simulink model "mpc_model_dual_module_allfreq"  (R2019a)
settings: Solver=FixedStepAuto  StartTime=0.0  StopTime=Tfinal  RelTol=1e-3
values from neighbouring files (symbols this model uses):
  A = [-0.0285 -0.0014; -0.0371 -0.1476]    [model.m]
  DCLINK_Cap = 1000e-12    (= 1e-09)    [mpc_model_parameters.m]    (also in mpc_model_parameters_dual_module.m = 0.001)
  FluxPM = MeanInducedVoltagePeak/(2*pi*100)    [mpc_model_parameters.m]    (also in mpc_model_parameters_dual_module.m)
  Inertia = 1e-2    (= 0.01)    [mpc_model_parameters.m]    (also in mpc_model_parameters_dual_module.m)
  iqrated = Trated/(1.5*PolePairs*FluxPM)    [mpc_model_parameters.m]    (also in mpc_model_parameters_dual_module.m)
  Ki = 8    [mpc_model_parameters_dual_module.m]
  Kp = 0.8    [mpc_model_parameters_dual_module.m]
  Ls = 3.5e-3    (= 0.0035)    [MPC_id_iq.m]    (also in mpc_model_parameters.m = 0.00351; mpc_model_parameters_dual_module.m = 0.00343)
  M1_FaultTime = 0.25    [mpc_model_parameters_dual_module.m]
  M2_FaultTime = 20    [mpc_model_parameters_dual_module.m]
  MeanLd = (1/12)*(Module1Phase_A_Ld+Module1Phase_B_Ld+Module1Phase_C_Ld+     Module2Phase_A_Ld+Module2Phase_B_Ld+Module2Phase_C_Ld+     Module3Phase_A_Ld+Module3Phase_B_Ld+Module3Phase_C_Ld+     Module4Phase_A_Ld+Module4Phase_B_Ld+Module4Phase_C_Ld)    [mpc_model_parameters.m]    (also in mpc_model_parameters_dual_module.m)
  MeanLq = (1/12)*(Module1Phase_A_Lq+Module1Phase_B_Lq+Module1Phase_C_Lq+     Module2Phase_A_Lq+Module2Phase_B_Lq+Module2Phase_C_Lq+     Module3Phase_A_Lq+Module3Phase_B_Lq+Module3Phase_C_Lq+     Module4Phase_A_Lq+Module4Phase_B_Lq+Module4Phase_C_Lq)    [mpc_model_parameters.m]    (also in mpc_model_parameters_dual_module.m)
  PI_Frequency = 5000    [mpc_model_parameters_dual_module.m]
  PI_Sat = iqrated*2    [mpc_model_parameters_dual_module.m]
  PI_Ts = 1/PI_Frequency    (= 0.0002)    [mpc_model_parameters_dual_module.m]
  PolePairs = 10    [mpc_model_parameters.m]    (also in mpc_model_parameters_dual_module.m)
  RefModeSelection = 1    [mpc_model_parameters_dual_module.m]
  Rin = 1e-3    (= 0.001)    [mpc_model_parameters.m]    (also in mpc_model_parameters_dual_module.m)
  Rs = 0.531    [Loss_Distribution.m]    (also in MPC_id_iq.m; mpc_model_parameters.m = 0.321; mpc_model_parameters_dual_module.m = 0.539)
  Sampling_time = 1e-6    (= 1e-06)    [mpc_model_parameters.m]    (also in mpc_model_parameters_dual_module.m)
  SpeedRef1 = 50    [mpc_model_parameters.m]    (also in mpc_model_parameters_dual_module.m = 35)
  SpeedRef2 = 100    [mpc_model_parameters.m]    (also in mpc_model_parameters_dual_module.m = 35)
  SpeedRefUpdateTime = 0.25    [mpc_model_parameters.m]    (also in mpc_model_parameters_dual_module.m = 1.75)
  Tload1 = 5    [mpc_model_parameters.m]    (also in mpc_model_parameters_dual_module.m = 30)
  Tload2 = 10    [mpc_model_parameters.m]    (also in mpc_model_parameters_dual_module.m = 63.6619772368)
  TloadUpdateTime = 0.5    [mpc_model_parameters.m]    (also in mpc_model_parameters_dual_module.m)
  Vdc = 50    [mpc_model_parameters.m]    (also in mpc_model_parameters_dual_module.m = 40)
  Vin = Vdc + Rin*(Pout/Vdc)    (= 50.04)    [mpc_model_parameters.m]    (also in mpc_model_parameters_dual_module.m = 40.05)
  ViscousFriction = 1e-3    (= 0.001)    [mpc_model_parameters.m]    (also in mpc_model_parameters_dual_module.m)
undefined symbols (not defined in the file or in its folder): DiscIntNeverNeededParam
libraries: powerlib x27, dspsigops x21, dspswit3 x19, powerlib_meascontrol x10, fl_lib x5, simulink x4, nesl_utility x3, sdl_lib x1
(part 2 of 3)

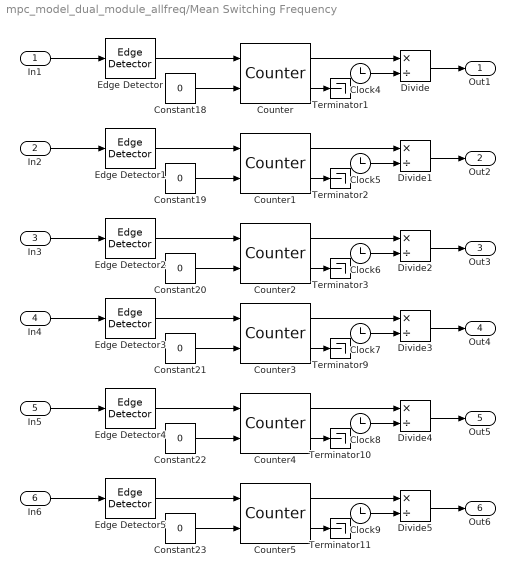
== system mpc_model_dual_module_allfreq/Mean Switching Frequency ==
  In1 : Inport
  In2 : Inport  Port=2
  In3 : Inport  Port=3
  In4 : Inport  Port=4
  In5 : Inport  Port=5
  In6 : Inport  Port=6
  Clock{4..9} (6 alike) : Clock
  Constant{18..23} (6 alike) : Constant  Value=0
  Counter{,1..5} (6 alike) : dspswit3/Counter  Direction=Up  CountEvent=Rising edge  CounterSize=User defined  MaxCount=9999999999999999999  InitialCount=0  Output=Count and Hit  HitValue=32  ResetInput=on  SamplesPerFrame=1  Ts=1  CntDtype=double  HitDtype=Logical
  Divide{,1..5} (6 alike) : Product  Inputs=*/
  Edge Detector{,1..5} (6 alike) : dspswit3/Edge Detector  InputProcessing=Columns as channels (frame based)
      settings: SourceProductName=DSP System Toolbox  SourceProductBaseCode=DS
  Terminator{1..3,9..11} (6 alike) : Terminator
  Out1 : Outport
  Out2 : Outport  Port=2
  Out3 : Outport  Port=3
  Out4 : Outport  Port=4
  Out5 : Outport  Port=5
  Out6 : Outport  Port=6
  wires:
  Counter5/2 -> Terminator11/1
  Divide2/1 -> Out3/1
  Clock8/1 -> Divide4/2
  Counter1/1 -> Divide1/1
  Constant22/1 -> Counter4/2
  Edge Detector5/1 -> Counter5/1
  Counter/2 -> Terminator1/1
  Edge Detector/1 -> Counter/1
  Counter5/1 -> Divide5/1
  Edge Detector2/1 -> Counter2/1
  Edge Detector4/1 -> Counter4/1
  Clock7/1 -> Divide3/2
  Counter4/2 -> Terminator10/1
  Constant19/1 -> Counter1/2
  Counter2/2 -> Terminator3/1
  Clock9/1 -> Divide5/2
  Constant20/1 -> Counter2/2
  Divide5/1 -> Out6/1
  Constant23/1 -> Counter5/2
  Edge Detector1/1 -> Counter1/1
  Counter4/1 -> Divide4/1
  Clock5/1 -> Divide1/2
  Counter3/2 -> Terminator9/1
  Counter2/1 -> Divide2/1
  Constant18/1 -> Counter/2
  In6/1 -> Edge Detector5/1
  Constant21/1 -> Counter3/2
  Counter3/1 -> Divide3/1
  Edge Detector3/1 -> Counter3/1
  Divide3/1 -> Out4/1
  Counter1/2 -> Terminator2/1
  In5/1 -> Edge Detector4/1
  Clock6/1 -> Divide2/2
  Divide/1 -> Out1/1
  Counter/1 -> Divide/1
  Clock4/1 -> Divide/2
  Divide4/1 -> Out5/1
  In4/1 -> Edge Detector3/1
  In2/1 -> Edge Detector1/1
  Divide1/1 -> Out2/1
  In3/1 -> Edge Detector2/1
  In1/1 -> Edge Detector/1

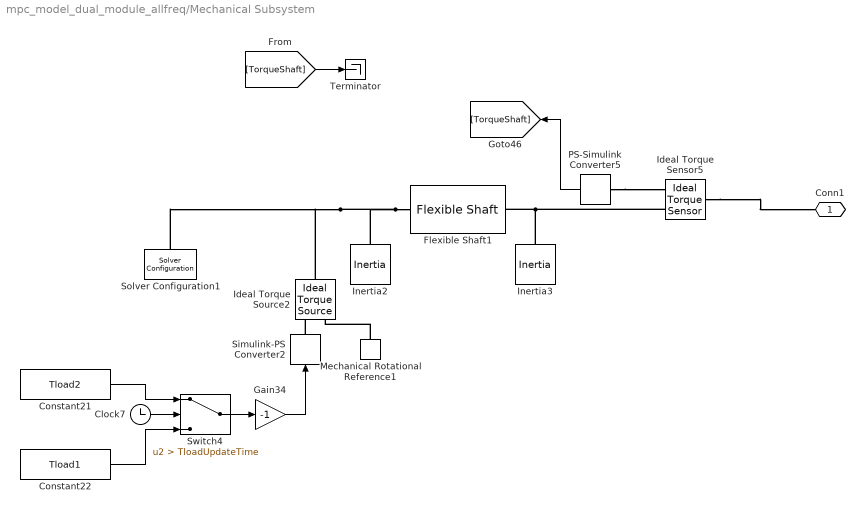
== system mpc_model_dual_module_allfreq/Mechanical Subsystem ==
  Clock7 : Clock
  Constant21 : Constant  Value=Tload2
  Constant22 : Constant  Value=Tload1
  Flexible Shaft1 : sdl_lib/Couplings & Drives/Flexible Shaft  modelTransverse=simscape.enum.onoff.off  parameterization=1  n_segments=10  shaft_stiffness=MechanicalShaftStiffness N*m/rad  shaft_inertia=MechanicalShaftInertia kg*m^2  length=1 m  eiIN=5e5 m^4*Pa  rhoaIN=19 kg/m  shaft_construction=1  diameter_outer=0.075 m  diameter_inner=0.05 m  density=7.8e+3 kg/m^3  shear_modulus=7.93e+10 Pa  elastic_modulus=200e9 Pa  damping_ratio=MechanicalShaftDampingRatio  mu_visc=[ 0 0 ] N*m/(rad/s)  boundaryC=sdl.enum.shaftSupport.clamp  KtransC_row=[10000000, 10000000] N/m  KrotC_row=[10000000, 10000000] N*m/rad  boundaryR=sdl.enum.shaftSupport.clamp  KtransR_row=[10000000, 10000000] N/m  KrotR_row=[10000000, 10000000] N*m/rad  alpha=10 1/s  beta=1e-8 s  d_bearing_trans=[0, 0] N/(m/s)  d_bearing_rotation=[0, 0] N*m/(rad/s)  noDisk=sdl.enum.shaftDisks.none  zDisk=0.5 m  mDiskIN=2 kg  IdDiskIN=0.025 kg*m^2  IpDiskIN=0.050 kg*m^2  offsetMR=[.01, .01] m*kg  offsetMassLocation=[.33, .67] m  offsetMR_initialAngleIN=[0, pi] rad  AnalysisMethod=sdl.enum.bendingAnalysisMethod.LumpedMass  ModeInputMethod=sdl.enum.modeInputMethod.SimscapeDetermined  numModesIn=6  OmegaNom=100 rpm  dw=5 rad/s  dwRefineFactor=1e-4  wMax=50000 rad/s  dz=0.01 m  userMode_w=[162, 162, 649, 649, 1460, 1460, 2596, 2596] rad/s  userMode_z=[0 : 0.1 : 1] m  userMode_shape=[0, 0, 0, 0, 0, 0, 0, 0, 0, 0, 0, 0, 0, 0, 0, 0; .309, 0, 0, .309, .5878, 0, 0, .5878, .809, 0, 0, .809, .9511, 0, 0, .9511; .5878, 0, 0, .5878, .9511, 0, 0, .9511, .9511, 0, 0, .9511, .5878, 0, 0, .5878; .809, 0, 0, .809, .9511, 0, 0, .9511, .309, 0, 0, .309, -.5878, 0, 0, -.5878; .9511, 0, 0, .9511, .5878, 0, 0, .5878, -.5878, 0, 0, -.5878, -.9511, 0, 0, -.9511; 1, 0, 0, 1, 0, 0, 0, 0, -1, 0, 0, -1, 0, 0, 0, 0; .9511, 0, 0, .9511, -.5878, 0, 0, -.5878, -.5878, 0, 0, -.5878, .9511, 0, 0, .9511; .809, 0, 0, .809, -.9511, 0, 0, -.9511, .309, 0, 0, .309, .5878, 0, 0, .5878; .5878, 0, 0, .5878, -.9511, 0, 0, -.9511, .9511, 0, 0, .9511, -.5878, 0, 0, -.5878; .309, 0, 0, .309, -.5878, 0, 0, -.5878, .809, 0, 0, .809, -.9511, 0, 0, -.9511; 0, 0, 0, 0, 0, 0, 0, 0, 0, 0, 0, 0, 0, 0, 0, 0]  initial_deflection=0 rad  initial_velocity=0 rpm
      settings: SourceProductName=Simscape Driveline  SourceProductBaseCode=LD
  Gain34 : Gain  Gain=-1
  Ideal Torque Sensor5 : fl_lib/Mechanical/Mechanical Sensors/Ideal Torque Sensor
  Ideal Torque Source2 : fl_lib/Mechanical/Mechanical Sources/Ideal Torque Source
  Inertia2 : fl_lib/Mechanical/Rotational Elements/Inertia  inertia=MechanicalInertia1 kg*m^2  w_specify=off  w_priority=High  w=0 rad/s  w_nominal_specify=off  w_nominal_unit=rad/s  w_nominal_value=1  t_specify=off  t_priority=None  t=0 N*m  t_nominal_specify=off  t_nominal_unit=N*m  t_nominal_value=1
  Inertia3 : fl_lib/Mechanical/Rotational Elements/Inertia  inertia=MechanicalInertia1 kg*m^2  w_specify=off  w_priority=High  w=0 rad/s  w_nominal_specify=off  w_nominal_unit=rad/s  w_nominal_value=1  t_specify=off  t_priority=None  t=0 N*m  t_nominal_specify=off  t_nominal_unit=N*m  t_nominal_value=1
  Mechanical Rotational Reference1 : fl_lib/Mechanical/Rotational Elements/Mechanical Rotational Reference
  PS-Simulink Converter5 : nesl_utility/PS-Simulink Converter  PhysicalDomain=network_engine_domain  SubClassName=ps_output  LeftPortType=input  RightPortType=output  PseudoPeriodic=off  Frequencies=[]  Unit=1  AffineConversion=off
  Simulink-PS Converter2 : nesl_utility/Simulink-PS Converter  PhysicalDomain=network_engine_domain  SubClassName=ps_input  LeftPortType=input  RightPortType=output  PseudoPeriodic=off  Frequencies=[]  NoiseDistribution=none  NoiseParameters=[]  Unit=1  AffineConversion=off  FilteringAndDerivatives=zero  SimscapeFilterOrder=1  InputFilterTimeConstant=0.001  UdotUserProvided=1
  Solver Configuration1 : nesl_utility/Solver Configuration  PhysicalDomain=network_engine_domain  SubClassName=solver  LeftPortType=input  RightPortType=generic  Tones=[]  Harmonics=[]  SimulateNoise=off  Profile=off  UseLocalSampling=off  EnableSwitchedLinearOptims=on  FrequencyDomain=off  UseCCode=off  RelTol=0.001  AbsTol=1e-06  MinStep=1e-09  ToWorkspace=off  RevertToSquareIcSolve=off  NumHomotopyIterations=100  PhasorMode=off  PhasorModeNumHarmonics=1  DoDC=off  ResidualTolerance=1e-09  UseLocalSolver=off  LocalSolverChoice=NE_BACKWARD_EULER_ADVANCER  LocalSolverSampleTime=0.001  DoFixedCost=off  MaxNonlinIter=3  MaxModeIter=2  LinearAlgebra=Sparse  EquationFormulation=NE_TIME_EF  DelaysMemoryBudget=1024  AutomaticFiltering=on  FilteringTimeConstant=0.001  PartitionStorageMethod=AS_NEEDED  PartitionMemoryBudget=1024  PartitionMethod=FAST
  Switch4 : Switch  Criteria=u2 > Threshold  Threshold=TloadUpdateTime
  Terminator : Terminator
  Conn1 : PMIOPort  Side=Left
  wires:
  Clock7/1 -> Switch4/2
  Constant21/1 -> Switch4/1
  Gain34/1 -> Simulink-PS Converter2/1
  PS-Simulink Converter5/1 -> [TorqueShaft]
  Switch4/1 -> Gain34/1
  Constant22/1 -> Switch4/3
  [TorqueShaft] -> Terminator/1
  connections:
  Flexible Shaft1/LConn1 -- Inertia2/LConn1 -- Solver Configuration1/RConn1 -- Ideal Torque Source2/LConn1
  Ideal Torque Sensor5/LConn1 -- Conn1/RConn1
  Ideal Torque Sensor5/RConn1 -- Inertia3/LConn1 -- Flexible Shaft1/RConn1
  Simulink-PS Converter2/RConn1 -- Ideal Torque Source2/RConn1
  Mechanical Rotational Reference1/LConn1 -- Ideal Torque Source2/RConn2
  PS-Simulink Converter5/LConn1 -- Ideal Torque Sensor5/RConn2

== matlab function mpc_model_dual_module_allfreq/MATLAB Function3 ==
  data: M1_copperloss output; M2_copperloss output; M1_magneticloss output; M2_magneticloss output; iqref input; M1_iqref output; M1_idref output; M2_iqref output; M2_idref output; Rs input; M1_FaultTime input; clock input; Ls input; ElectricalAngle input; M1_iqref_prev input; M1_idref_prev input; M2_iqref_prev input; M2_idref_prev input; M1_Iq_Opt_Proportional_prev input; M1_Id_Opt_Proportional_prev input; M2_Iq_Opt_Proportional_prev input; M2_Id_Opt_Proportional_prev input; ElectricalSpeed input; FluxPM input; pulse input; M1_Iq_Opt_Proportional output; M1_Id_Opt_Proportional output; M2_Iq_Opt_Proportional output; M2_Id_Opt_Proportional output; weight output; M1_lossfactor output; M2_lossfactor output; M1_lossfactor_prev input; M2_lossfactor_prev input
function [M1_copperloss,M2_copperloss,M1_magneticloss,M2_magneticloss,M1_iqref, M1_idref, M2_iqref, M2_idref,M1_Iq_Opt_Proportional,M1_Id_Opt_Proportional,M2_Iq_Opt_Proportional,M2_Id_Opt_Proportional,weight,M1_lossfactor,M2_lossfactor] = fcn(iqref, Rs, M1_FaultTime, clock, Ls, ElectricalAngle,M1_iqref_prev, M1_idref_prev, M2_iqref_prev, M2_idref_prev, M1_Iq_Opt_Proportional_prev, M1_Id_Opt_Proportional_prev, M2_Iq_Opt_Proportional_prev, M2_Id_Opt_Proportional_prev, ElectricalSpeed, FluxPM, pulse,M1_lossfactor_prev,M2_lossfactor_prev)

iqrated = 11.7362;
optimizationstep = 100;

% M2_iqref = iqref-M1_iqs;
M1_iqref_hyp = zeros(1,optimizationstep+1);
M2_iqref_hyp = zeros(1,optimizationstep+1);
M1_idref_hyp = zeros(1,optimizationstep+1);
M2_idref_hyp = zeros(1,optimizationstep+1);

M1_copper_loss = zeros(1,optimizationstep+1);
M2_copper_loss = zeros(1,optimizationstep+1);
M1_magnetic_loss = zeros(1,optimizationstep+1);
M2_magnetic_loss = zeros(1,optimizationstep+1);
Total_copper_loss = zeros(1,optimizationstep+1);
Total_magnetic_loss = zeros(1,optimizationstep+1);
cost = zeros(1,optimizationstep+1);
MinLossIndex = 0;

M1_Possible_Iq = zeros(1,optimizationstep+1);
M1_Possible_Id = zeros(1,optimizationstep+1);
M2_Possible_Iq = zeros(1,optimizationstep+1);
M2_Possible_Id = zeros(1,optimizationstep+1);

M1_magneticloss = 0;
M2_magneticloss = 0;

M1_copperloss = 0;
M2_copperloss = 0;

cfe = 1.15;
lambda = 1.15;
weight = 1;

% if(clock>M1_FaultTime)
if(iqref>iqrated)
    M1_lossfactor = 1;
    M2_lossfactor = 1;    
else
    M1_lossfactor = 1;
    M2_lossfactor = 1;    
end



% % % if(iqref>iqrated)
% % %     M1_lossfactor = 3;
% % %     M2_lossfactor = 2;
% % % else
% % %     M1_lossfactor = 1;
% % %     M2_lossfactor = 1;
% % % end

if(pulse==1)
    for i = 0:optimizationstep
        if(clock>M1_FaultTime)
% % % % %             M1_Possible_Iq(i+1) =  2/3*sin(2*pi/3)*(1+cos(2*ElectricalAngle+pi));
% % % % %             M1_Possible_Id(i+1) =  2/3*sin(2*pi/3)*(sin(2*ElectricalAngle+pi));
% % % % %             M2_Possible_Iq(i+1) = 1;
% % % % %             M2_Possible_Id(i+1) = 0;
            if(iqref>iqrated)
                M1_Possible_Iq(i+1) =  2*2/3*sin(2*pi/3)*(1+cos(2*ElectricalAngle+pi));
                M1_Possible_Id(i+1) =  2*2/3*sin(2*pi/3)*(sin(2*ElectricalAngle+pi));
                M2_Possible_Iq(i+1) = 1;
                M2_Possible_Id(i+1) = 0;
            else
                M1_Possible_Iq(i+1) =  1*2/3*sin(2*pi/3)*(1+cos(2*ElectricalAngle+pi));
                M1_Possible_Id(i+1) =  1*2/3*sin(2*pi/3)*(sin(2*ElectricalAngle+pi));
                M2_Possible_Iq(i+1) = 1;
                M2_Possible_Id(i+1) = 0;
            end
        else
            M1_Possible_Iq(i+1) = 1;
            M1_Possible_Id(i+1) = 0;
            M2_Possible_Iq(i+1) = 1;
            M2_Possible_Id(i+1) = 0;
        end
        
%         if(clock>M1_FaultTime)
            M1_iqref_hyp(i+1) = (1/optimizationstep*i)*iqref*M1_Possible_Iq(i+1);
            M1_idref_hyp(i+1) = (1/optimizationstep*i)*iqref*M1_Possible_Id(i+1);

            M2_iqref_hyp(i+1) = iqref - M1_iqref_hyp(i+1);
            if(iqref>iqrated)
%                weight = 4.2605;
                 weight = abs(iqrated-M1_iqref_hyp(i+1))/iqrated/10;
            else
%                weight = 1;
            end
            

            
            loss_protection  = 0;
            
            if(M2_iqref_hyp(i+1)>1.5*iqrated)
%                 loss_protection = 100;
            end
            weight = 1;
            
%             M1_lossfactor = 2/3;
%             M2_lossfactor = 1;

            
%         else
%             M1_iqref_hyp(i+1) = (1/optimizationstep*i)*iqref;
%             M2_iqref_hyp(i+1) = (1-1/optimizationstep*i)*iqref;
%             
%         end
        
        M1_d_axis_flux = Ls*M1_idref_hyp(i+1)+FluxPM;
        M1_q_axis_flux = Ls*M1_iqref_hyp(i+1);
        M2_d_axis_flux = Ls*M2_idref_hyp(i+1)+FluxPM;
        M2_q_axis_flux = Ls*M2_iqref_hyp(i+1);

        M1_copper_loss(i+1) = 1.5*Rs*(M1_iqref_hyp(i+1)^2+M1_idref_hyp(i+1)^2);
        M2_copper_loss(i+1) = 1.5*Rs*(M2_iqref_hyp(i+1)^2+M2_idref_hyp(i+1)^2);
        
%         M1_magnetic_loss(i+1) = cfe*power(abs(ElectricalSpeed),lambda)*(M1_d_axis_flux^2+M1_q_axis_flux^2);
%         M2_magnetic_loss(i+1) = cfe*power(abs(ElectricalSpeed),lambda)*(M2_d_axis_flux^2+M2_q_axis_flux^2);
        
        Total_magnetic_loss(i+1) = M1_magnetic_loss(i+1)+ M2_magnetic_loss(i+1);
%         Total_copper_loss(i+1) = M1_copper_loss(i+1)*weight+M2_copper_loss(i+1);
        Total_copper_loss(i+1) = M1_copper_loss(i+1)*M1_lossfactor_prev+M2_copper_loss(i+1)*M2_lossfactor_prev;
        
%         cost(i+1) = Total_copper_loss(i+1) + 0*Total_magnetic_loss(i+1) + loss_protection;    % +100000*(M1_idref_hyp(i+1)^2);%;+200000000000*(M1_idref_hyp(i+1)^2);
        cost(i+1) = Total_copper_loss(i+1);    % +100000*(M1_idref_hyp(i+1)^2);%;+200000000000*(M1_idref_hyp(i+1)^2);
        
        
    end
    
    [MinLossValue,MinLossIndex] = min(cost);
    if(clock>M1_FaultTime)
        M1_Iq_Opt_Proportional = iqref*0.5*2/7*(1+cos(2*ElectricalAngle+pi));
        M1_Id_Opt_Proportional = iqref*0.5*2/7*(sin(2*ElectricalAngle+pi));
        M2_Iq_Opt_Proportional = iqref*0.5*(5/7-2/7*cos(2*ElectricalAngle+pi));
        M2_Id_Opt_Proportional = 0;
    else
        M1_Iq_Opt_Proportional = iqref*0.5;
        M1_Id_Opt_Proportional = 0;
        M2_Iq_Opt_Proportional = iqref*0.5;
        M2_Id_Opt_Proportional = 0;
    end
    
    M1_iqref = M1_iqref_hyp(MinLossIndex);
    M1_idref = M1_idref_hyp(MinLossIndex);
    
    M2_iqref = M2_iqref_hyp(MinLossIndex);
    M2_idref = M2_idref_hyp(MinLossIndex);
    
%     if(M2_iqref>iqrated)
% %             M1_lossfactor = 2/3;
%         M2_lossfactor = M2_lossfactor_prev+0.01;
%     else
%         if(clock>M1_FaultTime)
%         M2_lossfactor = M2_lossfactor_prev-0.01;
%         end
%     end
%     
    M1_magneticloss = M1_magnetic_loss(MinLossIndex);
    M2_magneticloss = M2_magnetic_loss(MinLossIndex);
    
    M1_copperloss = M1_copper_loss(MinLossIndex);
    M2_copperloss = M2_copper_loss(MinLossIndex);

    
else
    M1_iqref = M1_iqref_prev;
    M1_idref = M1_idref_prev;
    
    M2_iqref = M2_iqref_prev;
    M2_idref = M2_idref_prev;
    
    M1_Iq_Opt_Proportional = M1_Iq_Opt_Proportional_prev;
    M1_Id_Opt_Proportional = M1_Id_Opt_Proportional_prev;
    M2_Iq_Opt_Proportional = M2_Iq_Opt_Proportional_prev;
    M2_Id_Opt_Proportional = M2_Id_Opt_Proportional_prev;    
    

    
end

== matlab function mpc_model_dual_module_allfreq/MATLAB Function ==
  data: d input; a output; q input; zero input; b output; c output; angle input
function [a,b,c] = fcn(d,q,zero,angle)

a = sin(angle)          *d  + cos(angle)        *q + 1*zero;
b = sin(angle-2*pi/3)   *d  + cos(angle-2*pi/3) *q + 1*zero;
c = sin(angle+2*pi/3)   *d  + cos(angle+2*pi/3) *q + 1*zero;

== matlab function mpc_model_dual_module_allfreq/M2 Prediction ==
  data: DutyA output; DutyB output; DutyC output; iqref input; idref input; IdMeasured input; IqMeasured input; Ls input; Rs input; PolePairs input; wref input; ShaftAngularSpeed input; ShaftAngularSpeed_prev input; FluxPM input; Vdc input; ElectricalAngle input; InterruptPulse input; DutyA_prev input; DutyB_prev input; DutyC_prev input; SimulationClock input; FaultOccuranceTime input; FswSelected_prev input; FswSelected output; IqRipplePrediction output; IqRipplePrediction_prev input; Speed_Error_prev input; Speed_Error output; Vds_Optimum output; Vqs_Optimum output; Vds_Optimum_prev input; Vqs_Optimum_prev input; fsw_phase input; M1_fsw input; M2_fsw_prev input; M1_int_moment input; M2_int_moment input; filter_out output; filter_out_prev input; IdPrediction_1_array output; IqPrediction_1_array output; IdPrediction_2_array output; IqPrediction_2_array output
function [DutyA, DutyB, DutyC, FswSelected, IqRipplePrediction,Speed_Error,Vds_Optimum,Vqs_Optimum,filter_out,IdPrediction_1_array,IqPrediction_1_array,IdPrediction_2_array,IqPrediction_2_array] = fcn(iqref,idref,IdMeasured, IqMeasured,  Ls, Rs,PolePairs,wref, ShaftAngularSpeed, ShaftAngularSpeed_prev, FluxPM,Vdc,ElectricalAngle,InterruptPulse,DutyA_prev, DutyB_prev, DutyC_prev, SimulationClock,FaultOccuranceTime,FswSelected_prev, IqRipplePrediction_prev,Speed_Error_prev,Vds_Optimum_prev,Vqs_Optimum_prev, fsw_phase, M1_fsw, M2_fsw_prev,M1_int_moment, M2_int_moment,filter_out_prev)
Ld = Ls;
Lq = Ls;
Iq_Rated = 11.7362; %this is the rated value of the IqMeasured



% cost = zeros(1,8);
% VdPrediction_1 = zeros(1,8);
% VqPrediction_1 = zeros(1,8);
% FswOptions = [5000; 10000; 15000; 20000; 25000; 30000; 35000; 40000];
FswMax = 10000;
FswOptions = 1000:1000:FswMax;
cost = zeros(1,numel(FswOptions));
% VdPrediction_1 = zeros(1,numel(FswOptions));
% VqPrediction_1 = zeros(1,numel(FswOptions));
Vd_est_1 = zeros(1,numel(FswOptions));
Vq_est_1 = zeros(1,numel(FswOptions));
% Vd_est_2 = zeros(1,numel(FswOptions));
% Vq_est_2 = zeros(1,numel(FswOptions));
VdPrediction_2 = zeros(1,numel(FswOptions));
VqPrediction_2 = zeros(1,numel(FswOptions));
IqRipplePredictionArray_1 = zeros(1,numel(FswOptions));
IqRipplePredictionArray_2 = zeros(1,numel(FswOptions));
VoltageDuring_T1_1 = zeros(1,numel(FswOptions));
VoltageDuring_T2_1 = zeros(1,numel(FswOptions));
VoltageDuring_T0_1 = zeros(1,numel(FswOptions));
VoltageDuring_T1_2 = zeros(1,numel(FswOptions));
VoltageDuring_T2_2 = zeros(1,numel(FswOptions));
VoltageDuring_T0_2 = zeros(1,numel(FswOptions));
MagnitudePrediction_1 = zeros(1,numel(FswOptions));
MagnitudePrediction_2 = zeros(1,numel(FswOptions));

SvpwmT1Prediction_1 =  zeros(1,numel(FswOptions));
SvpwmT2Prediction_1 =  zeros(1,numel(FswOptions));
SvpwmT0Prediction_1 =  zeros(1,numel(FswOptions));

SvpwmT1Prediction_2 =  zeros(1,numel(FswOptions));
SvpwmT2Prediction_2 =  zeros(1,numel(FswOptions));
SvpwmT0Prediction_2 =  zeros(1,numel(FswOptions));

ValfaPrediction_1 = zeros(1,numel(FswOptions)); 
VbetaPrediction_1 = zeros(1,numel(FswOptions)); 
ValfaPrediction_2 = zeros(1,numel(FswOptions)); 
VbetaPrediction_2 = zeros(1,numel(FswOptions)); 
maPrediction_1 = zeros(1,numel(FswOptions)); 
maPrediction_2 = zeros(1,numel(FswOptions));

IqDelta_Prediction_During_T1_1 =  zeros(1,numel(FswOptions));
IqDelta_Prediction_During_T2_1 =  zeros(1,numel(FswOptions));
IqDelta_Prediction_During_T0_1 =  zeros(1,numel(FswOptions));
IqDelta_Prediction_During_T1_2 =  zeros(1,numel(FswOptions));
IqDelta_Prediction_During_T2_2 =  zeros(1,numel(FswOptions));
IqDelta_Prediction_During_T0_2 =  zeros(1,numel(FswOptions));
VoltageVectorAnglePredictionMod_1 = zeros(1,numel(FswOptions));
VoltageVectorAnglePrediction_1 = zeros(1,numel(FswOptions));
VoltageVectorAnglePredictionMod_2 = zeros(1,numel(FswOptions));
VoltageVectorAnglePrediction_2 = zeros(1,numel(FswOptions));

IdPrediction_1_array = zeros(1,numel(FswOptions));
IqPrediction_1_array = zeros(1,numel(FswOptions));
IdPrediction_2_array = zeros(1,numel(FswOptions));
IqPrediction_2_array = zeros(1,numel(FswOptions));

Vd_Vq_Kp = 10;
Vd_Vq_Ki = 1;

MinimumCostValue = 1e20;
MinimumCostIndex = -1;

p1 = zeros(1,numel(FswOptions));
p2 = zeros(1,numel(FswOptions));
p3 = zeros(1,numel(FswOptions));
p4 = zeros(1,numel(FswOptions));
p5 = zeros(1,numel(FswOptions));
p6 = zeros(1,numel(FswOptions));


M1_Next_Int_Moment = M1_int_moment + 1/M1_fsw;

% IqRippleCoeff = 100000;
% IqRefCoeff = 10000;
% IdRefCoeff = 15;
% FswCoeff = 1250;
% FswCoeff = ones(1,numel(FswOptions))*1050;

IqRippleCoeff = 1000000;
IqRefCoeff = 1000000;
IdRefCoeff = 1000000;
% % FswCoeff = 2000;
% % FswInertiaCoeff = 500;
FswPhaseCoeff = 5000;

FswCoeff = 1250/10;
FswInertiaCoeff = 750;

M1fsw_M2fsw_PhaseDifference = M2_int_moment - M1_int_moment;


Iq_1_Method1 = 0;
Id_1_Method1 = 0;
Iq_2_Method1 = 0;
Id_2_Method1 = 0;
Kp = 0.35;
Ki = 50;
Ts_PI = 1/40000;
OptimizeForFsws = 0;
DifferentFswCost = 0;
if(FswSelected_prev<=0)
    FswSelected_prev = 1000;
end
% % % % % if(FswSelected_prev==1000)
% % % % %     OptimizeForFsws = 1:1:2;
% % % % % else if(FswSelected_prev==10000)
% % % % %      OptimizeForFsws = 9:1:10;
% % % % %     else
% % % % %         OptimizeForFsws = (FswSelected_prev/1000-1):1:(FswSelected_prev/1000+1);
% % % % %     end
% % % % % end

% % % % % % % % % if((FswSelected_prev==1000)||(FswSelected_prev==2000))
% % % % % % % % %     OptimizeForFsws = 1:1:5;
% % % % % % % % % else if((FswSelected_prev==10000)||(FswSelected_prev==9000))
% % % % % % % % %      OptimizeForFsws = 5:1:10;
% % % % % % % % %     else
% % % % % % % % %         OptimizeForFsws = (FswSelected_prev/1000-2):1:(FswSelected_prev/1000+2);
% % % % % % % % %     end
% % % % % % % % % end

if(FswSelected_prev==1000)
    OptimizeForFsws = 1:1:2;
else if(FswSelected_prev==10000)
     OptimizeForFsws = 9:1:10;
    else
        OptimizeForFsws = (FswSelected_prev/1000-1):1:(FswSelected_prev/1000+1);
    end
end


M1fsw_M2fsw_PhaseDifference_prediction = 0;


Speed_Error =  wref-ShaftAngularSpeed;
Speed_Error_RPM = Speed_Error/(2*pi)*60;

% deriv_speed = (ShaftAngularSpeed - ShaftAngularSpeed_prev)* FswSelected_prev;

if((abs(Speed_Error_RPM)>5)||(abs(filter_out_prev/100)>5))
    %         OptimizeForFsws(3) = 10;
    %         OptimizeForFsws(2) = 9;
    % IqRippleCoeff = 100000;
    IqRefCoeff = 1000000*100;
    IdRefCoeff = 1000000*100;
    FswPhaseCoeff = 0;
    % FswCoeff = 2500/5;
else
    IqRippleCoeff = 100000;
    IqRefCoeff = 1000000;
    IdRefCoeff = 1000000;
    FswPhaseCoeff = 5000;    
%     FswCoeff = 2000;
end


% y = y_prev + Kp*(u-u_prev)+Ts/2*Ki*(u+u_prev);
if(InterruptPulse==1)
    Speed_Error =  wref-ShaftAngularSpeed;
    Speed_Error_RPM =  Speed_Error/(2*pi)*60;
    
    
    filter_out = filter_out_prev + Speed_Error_RPM;
    filter_out = filter_out - filter_out/100;
        
%     iqref = iqref_prev + Kp*(Speed_Error-Speed_Error_prev)+Ts_PI/2*Ki*((Speed_Error+Speed_Error_prev));
% 
%     if(abs(iqref)>(2*Iq_Rated))
%         if(iqref>0)
%             iqref = (2*Iq_Rated);
%         else
%             iqref = -(2*Iq_Rated);
%         end
%     end
    for i = 1:numel(FswOptions)
%     for i = OptimizeForFsws(1):OptimizeForFsws(end)

        IdPrediction_1 = IdMeasured + (0.5/FswSelected_prev + 0.5/FswOptions(i))*(Vds_Optimum_prev/Ld-Rs/Ld*IdMeasured+Lq/Ld*PolePairs*ShaftAngularSpeed*IqMeasured);
        IqPrediction_1 = IqMeasured + (0.5/FswSelected_prev + 0.5/FswOptions(i))*(Vqs_Optimum_prev/Lq-Rs/Lq*IqMeasured-Ld/Lq*PolePairs*ShaftAngularSpeed*IdMeasured-FluxPM*PolePairs*ShaftAngularSpeed/Lq);
        
                
        IdPrediction_1_array(i) = IdPrediction_1;
        IqPrediction_1_array(i) = IqPrediction_1;

        M2_Next_Int_Moment = M2_int_moment + 1/FswOptions(i);
%         if(FswOptions(i) == M1_fsw)
%             if (((abs(M2_Next_Int_Moment-M1_Next_Int_Moment))*M1_fsw) > 0.74) && (((abs(M2_Next_Int_Moment-M1_Next_Int_Moment))*M1_fsw) < 0.76)
%                 
%             else
%                 
%                 FswCoeff(i) = 1250*3;
% %                 IqRippleCoeff = 100000;
%             end
%             DifferentFswCost = 0;            
%         else
%             FswCoeff(i) = 1250;
%             DifferentFswCost = 1500;
%             IqRippleCoeff = 100000;
%         end        
        
        Vd_Vq_Kp = Ls/(2)*FswOptions(i);
        Vd_Vq_Ki = Rs/Ls;
        
        Vd_est_1(i) = Vd_Vq_Kp * (idref-IdPrediction_1) * ( 1 + Vd_Vq_Ki / FswOptions(i) ) + IdMeasured - PolePairs*ShaftAngularSpeed*Ls*IqPrediction_1;
        Vq_est_1(i) = Vd_Vq_Kp * (iqref-IqPrediction_1) * ( 1 + Vd_Vq_Ki / FswOptions(i) ) + IqMeasured + PolePairs*ShaftAngularSpeed*(Ls*IdPrediction_1 + FluxPM);

        
     
        
        %% second prediction
        
%         M1fsw_M2fsw_PhaseDifference_prediction = - 1/M1_fsw + M1fsw_M2fsw_PhaseDifference + 1/FswOptions(i);        
        
        M1fsw_M2fsw_PhaseDifference_prediction = (M1fsw_M2fsw_PhaseDifference*FswOptions(i)-0.25)^2;
        
        MagnitudePrediction_2(i) = sqrt(Vd_est_1(i)^2+Vq_est_1(i)^2);
        
        ValfaPrediction_2(i) = sin(ElectricalAngle)*Vd_est_1(i)+cos(ElectricalAngle)*Vq_est_1(i);
        VbetaPrediction_2(i) =-cos(ElectricalAngle)*Vd_est_1(i)+sin(ElectricalAngle)*Vq_est_1(i);      
        
        VoltageVectorAnglePrediction_2(i) = atan2(VbetaPrediction_2(i),ValfaPrediction_2(i))+4*pi;%(PolePairs*ShaftAngularSpeed/FswOptions(i));
        VoltageVectorAnglePredictionMod_2(i) = mod(VoltageVectorAnglePrediction_2(i),pi/3);   
        
        maPrediction_2(i) = MagnitudePrediction_2(i)/(Vdc/sqrt(3)); 
        
        SvpwmT1Prediction_2(i) = (1/FswOptions(i))*maPrediction_2(i)*sin(pi/3-VoltageVectorAnglePredictionMod_2(i));
        SvpwmT2Prediction_2(i) = (1/FswOptions(i))*maPrediction_2(i)*sin(VoltageVectorAnglePredictionMod_2(i));
        SvpwmT0Prediction_2(i) = (1/FswOptions(i))-SvpwmT1Prediction_2(i)-SvpwmT2Prediction_2(i); 
        
        VoltageDuring_T1_2(i) = 2/3*Vdc-MagnitudePrediction_2(i);
        VoltageDuring_T2_2(i) = 2/3*Vdc-MagnitudePrediction_2(i);
        VoltageDuring_T0_2(i) = -MagnitudePrediction_2(i);
        
        IqDelta_Prediction_During_T1_2(i) = -VoltageDuring_T1_2(i)*SvpwmT1Prediction_2(i)/Ls;
        IqDelta_Prediction_During_T2_2(i) = -VoltageDuring_T2_2(i)*SvpwmT2Prediction_2(i)/Ls;
        IqDelta_Prediction_During_T0_2(i) = VoltageDuring_T0_2(i)*SvpwmT0Prediction_2(i)/Ls;        
        
        IqRipplePredictionArray_2(i) = IqDelta_Prediction_During_T1_2(i)+IqDelta_Prediction_During_T2_2(i)+IqDelta_Prediction_During_T0_2(i);
        
        IdPrediction_2 = IdPrediction_1 + (1/FswOptions(i))*(Vd_est_1(i)/Ld-Rs/Ld*IdPrediction_1+Lq/Ld*PolePairs*ShaftAngularSpeed*IqPrediction_1);
        IqPrediction_2 = IqPrediction_1 + (1/FswOptions(i))*(Vq_est_1(i)/Lq-Rs/Lq*IqPrediction_1-Ld/Lq*PolePairs*ShaftAngularSpeed*IdPrediction_1-FluxPM*PolePairs*ShaftAngularSpeed/Lq);                
        
        IdPrediction_2_array(i) = IdPrediction_2;
        IqPrediction_2_array(i) = IqPrediction_2;
        

        ProtectionConstant = 0;
        
        
% % %         cost(i) = M1fsw_M2fsw_PhaseDifference_prediction * 10000/4 + 0*50000*( abs(M1fsw_M2fsw_PhaseDifference_prediction) *  M1_fsw - .25)^2 + DifferentFswCost + 0*500*((FswOptions(i)-M1_fsw)/FswMax)^2+(IqRipplePredictionArray_2(i)/Iq_Rated)^2*IqRippleCoeff+IqRefCoeff*((iqref-IqPrediction_2)/Iq_Rated)^2+((idref-IdPrediction_2)/Iq_Rated)^2*IdRefCoeff+ProtectionConstant+FswOptions(i)/FswMax*FswCoeff(i);%+IqRipplePrediction_prev^2*100000000;
%         cost(i) = abs(M2_fsw_prev-FswOptions(i))/10000*FswInertiaCoeff + M1fsw_M2fsw_PhaseDifference_prediction*FswPhaseCoeff + (IqRipplePredictionArray_2(i)/Iq_Rated)^2*IqRippleCoeff+IqRefCoeff*((iqref-IqPrediction_2)/Iq_Rated)^2+((idref-IdPrediction_2)/Iq_Rated)^2*IdRefCoeff+ProtectionConstant+FswOptions(i)/FswMax*FswCoeff;
        
p1(i) = abs(M2_fsw_prev-FswOptions(i))/10000*FswInertiaCoeff ;
p2(i) = M1fsw_M2fsw_PhaseDifference_prediction*FswPhaseCoeff ;
p3(i) = (IqRipplePredictionArray_2(i)/Iq_Rated)^2*IqRippleCoeff;
p4(i) = IqRefCoeff*((iqref-IqPrediction_2)/Iq_Rated)^2;
p5(i) = ((idref-IdPrediction_2)/Iq_Rated)^2*IdRefCoeff;
p6(i) = FswOptions(i)/FswMax*FswCoeff;

cost(i) = p1(i)+p2(i)+p3(i)+p4(i)+p5(i)+p6(i);        
        if(cost(i)<MinimumCostValue)
            MinimumCostValue = cost(i);
            MinimumCostIndex = i;
        end
        
    end
    
%     [CostMinVal, MinimumCostIndex] = min(cost); 
    DutyA = 0;
    DutyB = 0;
    DutyC = 0;
    VdsOptimum_1 = VdPrediction_2(MinimumCostIndex);
    VqsOptimum_1 = VqPrediction_2(MinimumCostIndex);
    FswSelected = FswOptions(MinimumCostIndex);
    
    Iq_1_Method1 = IqPrediction_1_array(MinimumCostIndex);
    Id_1_Method1 = IdPrediction_1_array(MinimumCostIndex);

    Iq_2_Method1 = IqPrediction_2_array(MinimumCostIndex);
    Id_2_Method1 = IdPrediction_2_array(MinimumCostIndex);
    
    VoltageVectorAngleOptimum = VoltageVectorAnglePrediction_2(MinimumCostIndex);
    TswSelected = 1/FswSelected;
    
    Vds_Optimum = Vd_est_1(MinimumCostIndex);
    Vqs_Optimum = Vq_est_1(MinimumCostIndex);

    
    Svpwm_T1 = SvpwmT1Prediction_2(MinimumCostIndex);
    Svpwm_T2 = SvpwmT2Prediction_2(MinimumCostIndex);
    Svpwm_T0 = SvpwmT0Prediction_2(MinimumCostIndex);
    
    IqRipplePrediction = IqRipplePredictionArray_2(MinimumCostIndex);
    
    if (mod(VoltageVectorAngleOptimum, 2*pi)<=pi/3)&&(mod(VoltageVectorAngleOptimum, 2*pi)>=0)  % sector 1
        DutyA = (Svpwm_T1+Svpwm_T2+Svpwm_T0/2)/TswSelected;
        DutyB = (Svpwm_T2+Svpwm_T0/2)/TswSelected;
        DutyC = (Svpwm_T0/2)/TswSelected;
%         sectornumber = 1;
        return;
    end
    if (mod(VoltageVectorAngleOptimum, 2*pi)<=2*pi/3)&&(mod(VoltageVectorAngleOptimum, 2*pi)>=pi/3)  % sector 2
        DutyA = (Svpwm_T1+Svpwm_T0/2)/TswSelected;
        DutyB = (Svpwm_T1+Svpwm_T2+Svpwm_T0/2)/TswSelected;
        DutyC = (Svpwm_T0/2)/TswSelected;
%         sectornumber = 2;
        return;
    end
    if (mod(VoltageVectorAngleOptimum, 2*pi)<=pi)&&(mod(VoltageVectorAngleOptimum, 2*pi)>=2*pi/3)  % sector 3
        if(mod(VoltageVectorAngleOptimum, pi)==0)
            DutyA = (Svpwm_T0/2)/TswSelected;
            DutyB = (Svpwm_T1+Svpwm_T0/2)/TswSelected;
            DutyC = (Svpwm_T1+Svpwm_T2+Svpwm_T0/2)/TswSelected;
        else
            DutyA = (Svpwm_T0/2)/TswSelected;
            DutyB = (Svpwm_T1+Svpwm_T2+Svpwm_T0/2)/TswSelected;
            DutyC = (Svpwm_T2+Svpwm_T0/2)/TswSelected;
        end
%         sectornumber = 3;
        return;
    end
    if (mod(VoltageVectorAngleOptimum, 2*pi)<=4*pi/3)&&(mod(VoltageVectorAngleOptimum, 2*pi)>=pi)  % sector 4
        DutyA = (Svpwm_T0/2)/TswSelected;
        DutyB = (Svpwm_T1+Svpwm_T0/2)/TswSelected;
        DutyC = (Svpwm_T1+Svpwm_T2+Svpwm_T0/2)/TswSelected;
%         sectornumber = 4;
        return;
    end
    if (mod(VoltageVectorAngleOptimum, 2*pi)<=5*pi/3)&&(mod(VoltageVectorAngleOptimum, 2*pi)>=4*pi/3)  % sector 5
        DutyA = (Svpwm_T2+Svpwm_T0/2)/TswSelected;
        DutyB = (Svpwm_T0/2)/TswSelected;
        DutyC = (Svpwm_T1+Svpwm_T2+Svpwm_T0/2)/TswSelected;
%         sectornumber = 5;
        return;
    end
    if (mod(VoltageVectorAngleOptimum, 2*pi)<=2*pi)&&(mod(VoltageVectorAngleOptimum, 2*pi)>=5*pi/3)  % sector 6
        DutyA = (Svpwm_T1+Svpwm_T2+Svpwm_T0/2)/TswSelected;
        DutyB = (Svpwm_T0/2)/TswSelected;
        DutyC = (Svpwm_T1+Svpwm_T0/2)/TswSelected;
%         sectornumber = 6;
        return;
    end
    
else %switching pulse
%     iqref = iqref_prev;
    Speed_Error = Speed_Error_prev;
    FswSelected = FswSelected_prev;
    DutyA = DutyA_prev;
    DutyB = DutyB_prev;
    DutyC = DutyC_prev;
    IqRipplePrediction = IqRipplePrediction_prev;
    Vds_Optimum = Vds_Optimum_prev;
    Vqs_Optimum = Vqs_Optimum_prev;
    filter_out = filter_out_prev;
end

== matlab function mpc_model_dual_module_allfreq/MATLAB Function11 ==
  data: M1_id input; M1_iq input; M2_id input; M1_Torque output; M2_iq input; M2_Torque output
function [M1_Torque,M2_Torque] = fcn(M1_id, M1_iq, M2_id, M2_iq)

FluxPM = 0.18;
PolePairs = 10;
Ld = 3.5e-3;
M1_Torque = 3/2*PolePairs*M1_iq*(FluxPM+Ld*M1_id);

M2_Torque = 3/2*PolePairs*M2_iq*(FluxPM+Ld*M2_id);

== matlab function mpc_model_dual_module_allfreq/M1 Prediction ==
  data: DutyA output; DutyB output; DutyC output; iqref input; idref input; IdMeasured input; IqMeasured input; Ls input; Rs input; PolePairs input; wref input; ShaftAngularSpeed input; FluxPM input; Vdc input; ElectricalAngle input; InterruptPulse input; DutyA_prev input; DutyB_prev input; DutyC_prev input; SimulationClock input; FaultOccuranceTime input; FswSelected_prev input; FswSelected output; IqRipplePrediction output; IqRipplePrediction_prev input; Speed_Error_prev input; Speed_Error output; Vds_Optimum output; Vqs_Optimum output; Vds_Optimum_prev input; Vqs_Optimum_prev input; filter_out_prev input; filter_out output; IdPrediction_1_array output; IqPrediction_1_array output; IdPrediction_2_array output; IqPrediction_2_array output
function [DutyA, DutyB, DutyC, FswSelected, IqRipplePrediction,Speed_Error,Vds_Optimum,Vqs_Optimum,filter_out,IdPrediction_1_array,IqPrediction_1_array,IdPrediction_2_array,IqPrediction_2_array] = fcn(iqref,idref,IdMeasured, IqMeasured,  Ls, Rs,PolePairs,wref, ShaftAngularSpeed, FluxPM,Vdc,ElectricalAngle,InterruptPulse,DutyA_prev, DutyB_prev, DutyC_prev, SimulationClock,FaultOccuranceTime,FswSelected_prev, IqRipplePrediction_prev,Speed_Error_prev,Vds_Optimum_prev,Vqs_Optimum_prev,filter_out_prev)
Ld = Ls;
Lq = Ls;
Iq_Rated = 11.7362; %this is the rated value of the IqMeasured
% cost = zeros(1,8);
% VdPrediction_1 = zeros(1,8);
% VqPrediction_1 = zeros(1,8);
% FswOptions = [5000; 10000; 15000; 20000; 25000; 30000; 35000; 40000];
FswMax = 10000;
FswOptions = 1000:1000:FswMax;
cost = zeros(1,numel(FswOptions));
% VdPrediction_1 = zeros(1,numel(FswOptions));
% VqPrediction_1 = zeros(1,numel(FswOptions));
Vd_est_1 = zeros(1,numel(FswOptions));
Vq_est_1 = zeros(1,numel(FswOptions));
% Vd_est_2 = zeros(1,numel(FswOptions));
% Vq_est_2 = zeros(1,numel(FswOptions));
VdPrediction_2 = zeros(1,numel(FswOptions));
VqPrediction_2 = zeros(1,numel(FswOptions));
IqRipplePredictionArray_1 = zeros(1,numel(FswOptions));
IqRipplePredictionArray_2 = zeros(1,numel(FswOptions));
VoltageDuring_T1_1 = zeros(1,numel(FswOptions));
VoltageDuring_T2_1 = zeros(1,numel(FswOptions));
VoltageDuring_T0_1 = zeros(1,numel(FswOptions));
VoltageDuring_T1_2 = zeros(1,numel(FswOptions));
VoltageDuring_T2_2 = zeros(1,numel(FswOptions));
VoltageDuring_T0_2 = zeros(1,numel(FswOptions));
MagnitudePrediction_1 = zeros(1,numel(FswOptions));
MagnitudePrediction_2 = zeros(1,numel(FswOptions));

SvpwmT1Prediction_1 =  zeros(1,numel(FswOptions));
SvpwmT2Prediction_1 =  zeros(1,numel(FswOptions));
SvpwmT0Prediction_1 =  zeros(1,numel(FswOptions));

SvpwmT1Prediction_2 =  zeros(1,numel(FswOptions));
SvpwmT2Prediction_2 =  zeros(1,numel(FswOptions));
SvpwmT0Prediction_2 =  zeros(1,numel(FswOptions));

ValfaPrediction_1 = zeros(1,numel(FswOptions)); 
VbetaPrediction_1 = zeros(1,numel(FswOptions)); 
ValfaPrediction_2 = zeros(1,numel(FswOptions)); 
VbetaPrediction_2 = zeros(1,numel(FswOptions)); 
maPrediction_1 = zeros(1,numel(FswOptions)); 
maPrediction_2 = zeros(1,numel(FswOptions));

IqDelta_Prediction_During_T1_1 =  zeros(1,numel(FswOptions));
IqDelta_Prediction_During_T2_1 =  zeros(1,numel(FswOptions));
IqDelta_Prediction_During_T0_1 =  zeros(1,numel(FswOptions));
IqDelta_Prediction_During_T1_2 =  zeros(1,numel(FswOptions));
IqDelta_Prediction_During_T2_2 =  zeros(1,numel(FswOptions));
IqDelta_Prediction_During_T0_2 =  zeros(1,numel(FswOptions));
VoltageVectorAnglePredictionMod_1 = zeros(1,numel(FswOptions));
VoltageVectorAnglePrediction_1 = zeros(1,numel(FswOptions));
VoltageVectorAnglePredictionMod_2 = zeros(1,numel(FswOptions));
VoltageVectorAnglePrediction_2 = zeros(1,numel(FswOptions));

IdPrediction_1_array = zeros(1,numel(FswOptions));
IqPrediction_1_array = zeros(1,numel(FswOptions));
IdPrediction_2_array = zeros(1,numel(FswOptions));
IqPrediction_2_array = zeros(1,numel(FswOptions));

p1 = zeros(1,numel(FswOptions));
p2 = zeros(1,numel(FswOptions));
p3 = zeros(1,numel(FswOptions));
p4 = zeros(1,numel(FswOptions));
p5 = zeros(1,numel(FswOptions));



Vd_Vq_Kp = 10;
Vd_Vq_Ki = 1;

MinimumCostValue = 1e20;
MinimumCostIndex = -1;

% IqRippleCoeff = 100000;
% IqRefCoeff = 10000;
% IdRefCoeff = 15;
% FswCoeff = 1250;

IqRippleCoeff = 100000;
IqRefCoeff = 1000000;
IdRefCoeff = 1000000;
FswCoeff = 1250;
FswInertiaCoeff = 750;


Iq_1_Method1 = 0;
Id_1_Method1 = 0;
Iq_2_Method1 = 0;
Id_2_Method1 = 0;
Kp = 0.35;
Ki = 50;
Ts_PI = 1/40000;
OptimizeForFsws = 0;
if(FswSelected_prev<=0)
    FswSelected_prev = 1000;
end
% % % % % % % % if((FswSelected_prev==1000)||(FswSelected_prev==2000))
% % % % % % % %     OptimizeForFsws = 1:1:5;
% % % % % % % % else if((FswSelected_prev==10000)||(FswSelected_prev==9000))
% % % % % % % %      OptimizeForFsws = 5:1:10;
% % % % % % % %     else
% % % % % % % %         OptimizeForFsws = (FswSelected_prev/1000-2):1:(FswSelected_prev/1000+2);
% % % % % % % %     end
% % % % % % % % end
if(FswSelected_prev==1000)
    OptimizeForFsws = 1:1:2;
else if(FswSelected_prev==10000)
     OptimizeForFsws = 9:1:10;
    else
        OptimizeForFsws = (FswSelected_prev/1000-1):1:(FswSelected_prev/1000+1);
    end
end

Speed_Error =  wref-ShaftAngularSpeed;
Speed_Error_RPM = Speed_Error/(2*pi)*60;

% deriv_speed = (ShaftAngularSpeed - ShaftAngularSpeed_prev)* FswSelected_prev;

if((abs(Speed_Error_RPM)>5)||(abs(filter_out_prev/100)>5))
    %         OptimizeForFsws(3) = 10;
    %         OptimizeForFsws(2) = 9;
    % IqRippleCoeff = 100000;
    IqRefCoeff = 1000000*100;
    IdRefCoeff = 1000000*100;
    % FswCoeff = 2500/5;
else
    IqRippleCoeff = 100000;
    IqRefCoeff = 1000000;
    IdRefCoeff = 1000000;
    FswCoeff = 1250;
end

% y = y_prev + Kp*(u-u_prev)+Ts/2*Ki*(u+u_prev);
if(InterruptPulse==1)
    Speed_Error =  wref-ShaftAngularSpeed;
    filter_out = filter_out_prev + Speed_Error_RPM;
    filter_out = filter_out - filter_out/100;    
%     iqref = iqref_prev + Kp*(Speed_Error-Speed_Error_prev)+Ts_PI/2*Ki*((Speed_Error+Speed_Error_prev));
% 
%     if(abs(iqref)>(2*Iq_Rated))
%         if(iqref>0)
%             iqref = (2*Iq_Rated);
%         else
%             iqref = -(2*Iq_Rated);
%         end
%     end
    for i = 1:numel(FswOptions)
%     for i = OptimizeForFsws(1):OptimizeForFsws(end)

        IdPrediction_1 = IdMeasured + (0.5/FswSelected_prev + 0.5/FswOptions(i))*(Vds_Optimum_prev/Ld-Rs/Ld*IdMeasured+Lq/Ld*PolePairs*ShaftAngularSpeed*IqMeasured);
        IqPrediction_1 = IqMeasured + (0.5/FswSelected_prev + 0.5/FswOptions(i))*(Vqs_Optimum_prev/Lq-Rs/Lq*IqMeasured-Ld/Lq*PolePairs*ShaftAngularSpeed*IdMeasured-FluxPM*PolePairs*ShaftAngularSpeed/Lq);
        
                
        IdPrediction_1_array(i) = IdPrediction_1;
        IqPrediction_1_array(i) = IqPrediction_1;
        
        Vd_Vq_Kp = Ls/(2)*FswOptions(i);
        Vd_Vq_Ki = Rs/Ls;
        
        Vd_est_1(i) = Vd_Vq_Kp * (idref-IdPrediction_1) * ( 1 + Vd_Vq_Ki / FswOptions(i) ) + IdMeasured - PolePairs*ShaftAngularSpeed*Ls*IqPrediction_1;
        Vq_est_1(i) = Vd_Vq_Kp * (iqref-IqPrediction_1) * ( 1 + Vd_Vq_Ki / FswOptions(i) ) + IqMeasured + PolePairs*ShaftAngularSpeed*(Ls*IdPrediction_1 + FluxPM);

        
     
        
        %% second prediction
        
        
        MagnitudePrediction_2(i) = sqrt(Vd_est_1(i)^2+Vq_est_1(i)^2);
        
        ValfaPrediction_2(i) = sin(ElectricalAngle)*Vd_est_1(i)+cos(ElectricalAngle)*Vq_est_1(i);
        VbetaPrediction_2(i) =-cos(ElectricalAngle)*Vd_est_1(i)+sin(ElectricalAngle)*Vq_est_1(i);      
        
        VoltageVectorAnglePrediction_2(i) = atan2(VbetaPrediction_2(i),ValfaPrediction_2(i))+4*pi;%(PolePairs*ShaftAngularSpeed/FswOptions(i));
        VoltageVectorAnglePredictionMod_2(i) = mod(VoltageVectorAnglePrediction_2(i),pi/3);   
        
        maPrediction_2(i) = MagnitudePrediction_2(i)/(Vdc/sqrt(3)); 
        
        if(SimulationClock>FaultOccuranceTime)
%             IqRefCoeff = 100;
            SvpwmT1Prediction_2(i) = (1/FswOptions(i))*maPrediction_2(i)*sin(mod(VoltageVectorAnglePrediction_2(i),pi));
            SvpwmT2Prediction_2(i) = 0;
            SvpwmT0Prediction_2(i) = (1/FswOptions(i))-SvpwmT1Prediction_2(i)-SvpwmT2Prediction_2(i);       
        else
            SvpwmT1Prediction_2(i) = (1/FswOptions(i))*maPrediction_2(i)*sin(pi/3-VoltageVectorAnglePredictionMod_2(i));
            SvpwmT2Prediction_2(i) = (1/FswOptions(i))*maPrediction_2(i)*sin(VoltageVectorAnglePredictionMod_2(i));
            SvpwmT0Prediction_2(i) = (1/FswOptions(i))-SvpwmT1Prediction_2(i)-SvpwmT2Prediction_2(i);    
        end  
        
        VoltageDuring_T1_2(i) = 2/3*Vdc-MagnitudePrediction_2(i);
        VoltageDuring_T2_2(i) = 2/3*Vdc-MagnitudePrediction_2(i);
        VoltageDuring_T0_2(i) = -MagnitudePrediction_2(i);
        
        IqDelta_Prediction_During_T1_2(i) = -VoltageDuring_T1_2(i)*SvpwmT1Prediction_2(i)/Ls;
        IqDelta_Prediction_During_T2_2(i) = -VoltageDuring_T2_2(i)*SvpwmT2Prediction_2(i)/Ls;
        IqDelta_Prediction_During_T0_2(i) = VoltageDuring_T0_2(i)*SvpwmT0Prediction_2(i)/Ls;        
        
        IqRipplePredictionArray_2(i) = IqDelta_Prediction_During_T1_2(i)+IqDelta_Prediction_During_T2_2(i)+IqDelta_Prediction_During_T0_2(i);
        
        IdPrediction_2 = IdPrediction_1 + (1/FswOptions(i))*(Vd_est_1(i)/Ld-Rs/Ld*IdPrediction_1+Lq/Ld*PolePairs*ShaftAngularSpeed*IqPrediction_1);
        IqPrediction_2 = IqPrediction_1 + (1/FswOptions(i))*(Vq_est_1(i)/Lq-Rs/Lq*IqPrediction_1-Ld/Lq*PolePairs*ShaftAngularSpeed*IdPrediction_1-FluxPM*PolePairs*ShaftAngularSpeed/Lq);                
        
        IdPrediction_2_array(i) = IdPrediction_2;
        IqPrediction_2_array(i) = IqPrediction_2;
        

        ProtectionConstant = 0;
%         cost(i) = FswInertiaCoeff*abs(FswSelected_prev-FswOptions(i))/FswMax+(IqRipplePredictionArray_2(i)/Iq_Rated)^2*IqRippleCoeff+IqRefCoeff*((iqref-IqPrediction_2)/Iq_Rated)^2+((idref-IdPrediction_2)/Iq_Rated)^2*IdRefCoeff+ProtectionConstant+FswOptions(i)/FswMax*FswCoeff;%+IqRipplePrediction_prev^2*100000000;

p1(i) = FswInertiaCoeff*abs(FswSelected_prev-FswOptions(i))/FswMax;
p2(i) = (IqRipplePredictionArray_2(i)/Iq_Rated)^2*IqRippleCoeff;
p3(i) = IqRefCoeff*((iqref-IqPrediction_2)/Iq_Rated)^2;
p4(i) = ((idref-IdPrediction_2)/Iq_Rated)^2*IdRefCoeff;
p5(i) = FswOptions(i)/FswMax*FswCoeff;
        cost(i) = p1(i) + p2(i) + p3(i) + p4(i) + p5(i);
        
        
        if(cost(i)<MinimumCostValue)
            MinimumCostValue = cost(i);
            MinimumCostIndex = i;
        end
        
    end
    
%     [CostMinVal, MinimumCostIndex] = min(cost);


    DutyA = 0;
    DutyB = 0;
    DutyC = 0;
    VdsOptimum_1 = VdPrediction_2(MinimumCostIndex);
    VqsOptimum_1 = VqPrediction_2(MinimumCostIndex);
    FswSelected = FswOptions(MinimumCostIndex);
    
    Iq_1_Method1 = IqPrediction_1_array(MinimumCostIndex);
    Id_1_Method1 = IdPrediction_1_array(MinimumCostIndex);

    Iq_2_Method1 = IqPrediction_2_array(MinimumCostIndex);
    Id_2_Method1 = IdPrediction_2_array(MinimumCostIndex);
    
    VoltageVectorAngleOptimum = VoltageVectorAnglePrediction_2(MinimumCostIndex);
    TswSelected = 1/FswSelected;
    
    Vds_Optimum = Vd_est_1(MinimumCostIndex);
    Vqs_Optimum = Vq_est_1(MinimumCostIndex);

    
    Svpwm_T1 = SvpwmT1Prediction_2(MinimumCostIndex);
    Svpwm_T2 = SvpwmT2Prediction_2(MinimumCostIndex);
    Svpwm_T0 = SvpwmT0Prediction_2(MinimumCostIndex);
    
    IqRipplePrediction = IqRipplePredictionArray_2(MinimumCostIndex);
    
    if(SimulationClock>FaultOccuranceTime)
        if (mod(VoltageVectorAngleOptimum, 2*pi)<=pi)  
            DutyB = (Svpwm_T1+Svpwm_T0/2)/TswSelected;
            DutyC = (Svpwm_T0/2)/TswSelected;
        else
            DutyC = (Svpwm_T1+Svpwm_T0/2)/TswSelected;
            DutyB = (Svpwm_T0/2)/TswSelected;
        end
        DutyA = 0;
        return;
    end        
    
    if (mod(VoltageVectorAngleOptimum, 2*pi)<=pi/3)&&(mod(VoltageVectorAngleOptimum, 2*pi)>=0)  % sector 1
        DutyA = (Svpwm_T1+Svpwm_T2+Svpwm_T0/2)/TswSelected;
        DutyB = (Svpwm_T2+Svpwm_T0/2)/TswSelected;
        DutyC = (Svpwm_T0/2)/TswSelected;
%         sectornumber = 1;
        return;
    end
    if (mod(VoltageVectorAngleOptimum, 2*pi)<=2*pi/3)&&(mod(VoltageVectorAngleOptimum, 2*pi)>=pi/3)  % sector 2
        DutyA = (Svpwm_T1+Svpwm_T0/2)/TswSelected;
        DutyB = (Svpwm_T1+Svpwm_T2+Svpwm_T0/2)/TswSelected;
        DutyC = (Svpwm_T0/2)/TswSelected;
%         sectornumber = 2;
        return;
    end
    if (mod(VoltageVectorAngleOptimum, 2*pi)<=pi)&&(mod(VoltageVectorAngleOptimum, 2*pi)>=2*pi/3)  % sector 3
        if(mod(VoltageVectorAngleOptimum, pi)==0)
            DutyA = (Svpwm_T0/2)/TswSelected;
            DutyB = (Svpwm_T1+Svpwm_T0/2)/TswSelected;
            DutyC = (Svpwm_T1+Svpwm_T2+Svpwm_T0/2)/TswSelected;
        else
            DutyA = (Svpwm_T0/2)/TswSelected;
            DutyB = (Svpwm_T1+Svpwm_T2+Svpwm_T0/2)/TswSelected;
            DutyC = (Svpwm_T2+Svpwm_T0/2)/TswSelected;
        end
%         sectornumber = 3;
        return;
    end
    if (mod(VoltageVectorAngleOptimum, 2*pi)<=4*pi/3)&&(mod(VoltageVectorAngleOptimum, 2*pi)>=pi)  % sector 4
        DutyA = (Svpwm_T0/2)/TswSelected;
        DutyB = (Svpwm_T1+Svpwm_T0/2)/TswSelected;
        DutyC = (Svpwm_T1+Svpwm_T2+Svpwm_T0/2)/TswSelected;
%         sectornumber = 4;
        return;
    end
    if (mod(VoltageVectorAngleOptimum, 2*pi)<=5*pi/3)&&(mod(VoltageVectorAngleOptimum, 2*pi)>=4*pi/3)  % sector 5
        DutyA = (Svpwm_T2+Svpwm_T0/2)/TswSelected;
        DutyB = (Svpwm_T0/2)/TswSelected;
        DutyC = (Svpwm_T1+Svpwm_T2+Svpwm_T0/2)/TswSelected;
%         sectornumber = 5;
        return;
    end
    if (mod(VoltageVectorAngleOptimum, 2*pi)<=2*pi)&&(mod(VoltageVectorAngleOptimum, 2*pi)>=5*pi/3)  % sector 6
        DutyA = (Svpwm_T1+Svpwm_T2+Svpwm_T0/2)/TswSelected;
        DutyB = (Svpwm_T0/2)/TswSelected;
        DutyC = (Svpwm_T1+Svpwm_T0/2)/TswSelected;
%         sectornumber = 6;
        return;
    end
    
else %switching pulse
%     iqref = iqref_prev;
    Speed_Error = Speed_Error_prev;
    FswSelected = FswSelected_prev;
    DutyA = DutyA_prev;
    DutyB = DutyB_prev;
    DutyC = DutyC_prev;
    IqRipplePrediction = IqRipplePrediction_prev;
    Vds_Optimum = Vds_Optimum_prev;
    Vqs_Optimum = Vqs_Optimum_prev;
    filter_out = filter_out_prev;    
end
